simulink model "drone_position_estimate_discrete"  (R2020b)
settings: Solver=VariableStepAuto  StartTime=0.0  StopTime=30  RelTol=1e-3
values from neighbouring files (symbols this model uses):
  at = [1;0;-9.98]    [run_drone_estimate.m]
  cov_an = 1*eye(3)    [run_drone_estimate.m]
  cov_aw = 1*eye(3)    [run_drone_estimate.m]
  cov_gps = .01*eye(3)    [run_drone_estimate.m]
  F_discrete = F_discrete + (aux/factorial(i))    [run_drone_estimate.m]
  g = [0;0;-9.98]    [run_drone_estimate.m]
  h = 1    [run_drone_estimate.m]
  H_discrete = H    [run_drone_estimate.m]
  L = lqe(F, G, H, Q, R)    [run_drone_estimate.m]
  p0 = zeros(3,1)    [run_drone_estimate.m]
  Rm = eye(3)    [run_drone_estimate.m]
  v0 = zeros(3,1)    [run_drone_estimate.m]
  x0_observer = zeros(n, 1)    [run_drone_estimate.m]
settings Model: Creator=lucas  LastModifiedBy=lucas

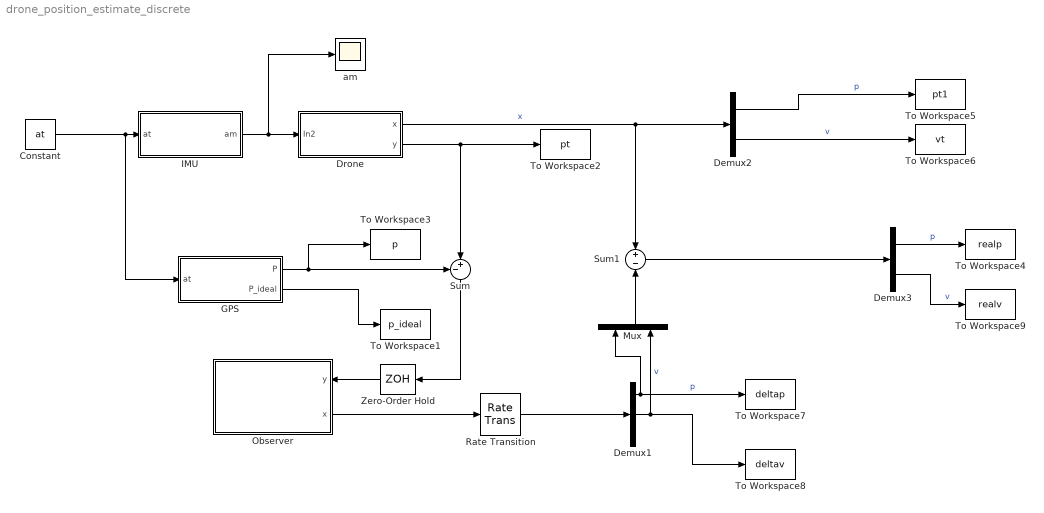
== system drone_position_estimate_discrete ==
  Constant : Constant  Value=at
  Demux1 : Demux  Outputs=3
  Demux2 : Demux  Outputs=2
  Demux3 : Demux  Outputs=2
  Drone : Subsystem
  GPS : Subsystem
  IMU : Subsystem
  Mux : Mux  Inputs=2
  Observer : Subsystem
      settings: PortSchema="{\"entries\":[{\"content\":{\"sides\":[{\"content\":{\"connectorIds\":[]},\"type\":\"ConnectorPlacement.EquallySpacedRectSide\",\"uuid\":\"b6dae28a-5485-44ef-84e6-2d14792229e7\"},{\"content\":{\"connectorIds\":[\"In1\",\"Out1\"],\"side\":\"RIGHT\"},\"type\":\"ConnectorPlacement.EquallySpacedRectSide\",\"uuid\":\"53a86c87-87d1-415f-9895-91b2b6ac7daf\"},{\"content\":{\"connectorIds\":[],\"side\":\"TOP\"},\"type\":\"ConnectorPlacement.EquallySpacedRectSide\",\"uuid\":\"c2916f3e-51bf-40f4-b6cd-eee6b60c38ec\"},{\"content\":{\"connectorIds\":[],\"side\":\"HIDDEN\"},\"type\":\"ConnectorPlacement.EquallySpacedRectSide\",\"uuid\":\"c85aafdf-e330-4d8d-a14a-206e12d7d836\"}]},\"type\":\"ConnectorPlacement.EquallySpacedConnector\",\"uuid\":\"08a8a426-31b9-42c2-8372-de3a4deaf2af\"}],\"packageUris\":[\"http://schema.mathworks.com/mf0/Connector/R2020b\"],\"version\":\"1.0\"}"
  Rate Transition : RateTransition  OutPortSampleTimeOpt=Inherit  OutPortSampleTimeMultiple=h_plant  OutPortSampleTime=h_plant
  Sum : Sum  Inputs=-+|
  Sum1 : Sum  Inputs=+|-
  To Workspace1 : ToWorkspace  VariableName=p_ideal  SaveFormat=Timeseries  SampleTime=-1
  To Workspace2 : ToWorkspace  VariableName=pt  SaveFormat=Timeseries  SampleTime=-1
  To Workspace3 : ToWorkspace  VariableName=p  SaveFormat=Timeseries  SampleTime=-1
  To Workspace4 : ToWorkspace  VariableName=realp  SaveFormat=Timeseries  SampleTime=-1
  To Workspace5 : ToWorkspace  VariableName=pt1  SaveFormat=Timeseries  SampleTime=-1
  To Workspace6 : ToWorkspace  VariableName=vt  SaveFormat=Timeseries  SampleTime=-1
  To Workspace7 : ToWorkspace  VariableName=deltap  SaveFormat=Timeseries  SampleTime=-1
  To Workspace8 : ToWorkspace  VariableName=deltav  SaveFormat=Timeseries  SampleTime=-1
  To Workspace9 : ToWorkspace  VariableName=realv  SaveFormat=Timeseries  SampleTime=-1
  Zero-Order Hold : ZeroOrderHold  SampleTime=h
  am : Scope
  wires:
  GPS/2(P_ideal) -> To Workspace1/1
  Constant/1 -> GPS/1(at), IMU/1(at)
  GPS/1(P) -> Sum/1, To Workspace3/1
  Demux1/1 -> Mux/1, To Workspace7/1  "p"
  IMU/1(am) -> am/1, Drone/1(In2)
  Demux1/2 -> Mux/2, To Workspace8/1  "v"
  Drone/1(x) -> Demux2/1, Sum1/1  "x"
  Demux2/2 -> To Workspace6/1  "v"
  Demux2/1 -> To Workspace5/1  "p"
  Drone/2(y) -> Sum/2, To Workspace2/1
  Zero-Order Hold/1 -> Observer/1(y)
  Sum/1 -> Zero-Order Hold/1
  Observer/1(x) -> Rate Transition/1
  Rate Transition/1 -> Demux1/1
  Sum1/1 -> Demux3/1
  Demux3/1 -> To Workspace4/1  "p"
  Demux3/2 -> To Workspace9/1  "v"
  Mux/1 -> Sum1/2

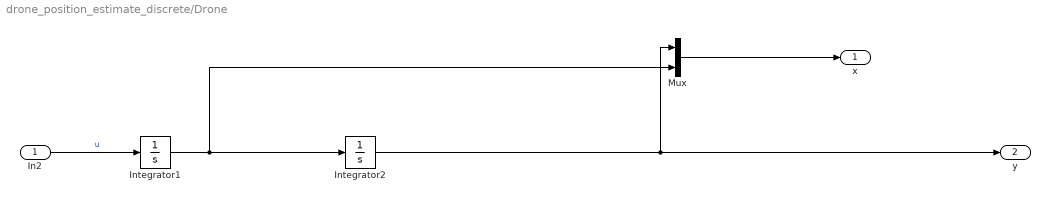
== system drone_position_estimate_discrete/Drone ==
  In2 : Inport
  Integrator1 : Integrator  InitialCondition=v0
  Integrator2 : Integrator  InitialCondition=p0
  Mux : Mux  Inputs=2
  x : Outport
  y : Outport  Port=2
  wires:
  In2/1 -> Integrator1/1  "u"
  Integrator1/1 -> Integrator2/1, Mux/2
  Integrator2/1 -> Mux/1, y/1
  Mux/1 -> x/1

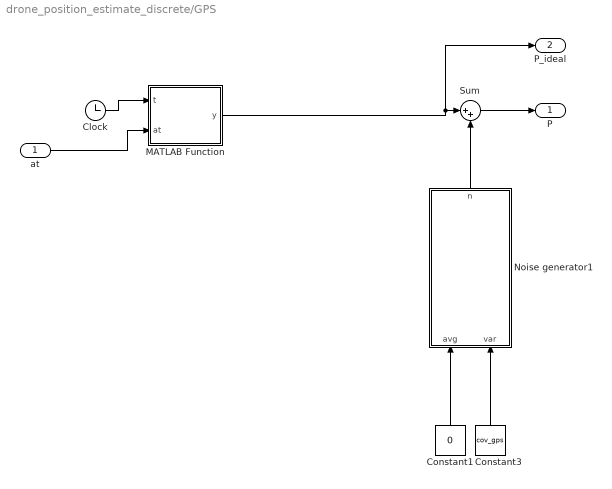
== system drone_position_estimate_discrete/GPS ==
  at : Inport
  Clock : Clock
  Constant1 : Constant  Value=0
  Constant3 : Constant  Value=cov_gps
  MATLAB Function : MATLAB Function  TreatAsAtomicUnit=on
  Noise generator1 : MATLAB Function  TreatAsAtomicUnit=on
  Sum : Sum  Inputs=|++
  P : Outport
  P_ideal : Outport  Port=2
  wires:
  Noise generator1/1(n) -> Sum/2
  Constant3/1 -> Noise generator1/2(var)
  Constant1/1 -> Noise generator1/1(avg)
  Sum/1 -> P/1
  Clock/1 -> MATLAB Function/1(t)
  MATLAB Function/1(y) -> P_ideal/1, Sum/1
  at/1 -> MATLAB Function/2(at)

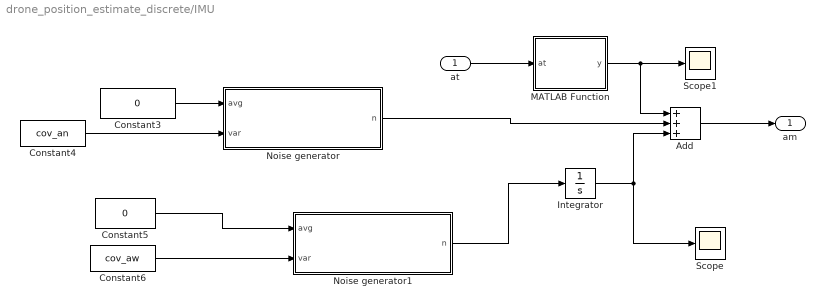
== system drone_position_estimate_discrete/IMU ==
  at : Inport
  Add : Sum  Inputs=+++
  Constant3 : Constant  Value=0  VectorParams1D=off
  Constant4 : Constant  Value=cov_an  VectorParams1D=off
  Constant5 : Constant  Value=0  VectorParams1D=off
  Constant6 : Constant  Value=cov_aw  VectorParams1D=off
  Integrator : Integrator
  MATLAB Function : MATLAB Function  TreatAsAtomicUnit=on
  Noise generator : MATLAB Function  TreatAsAtomicUnit=on
  Noise generator1 : MATLAB Function  TreatAsAtomicUnit=on
  Scope : Scope
  Scope1 : Scope
  am : Outport
  wires:
  Add/1 -> am/1
  Integrator/1 -> Scope/1, Add/3
  MATLAB Function/1(y) -> Scope1/1, Add/1
  Constant3/1 -> Noise generator/1(avg)
  Constant4/1 -> Noise generator/2(var)
  Noise generator/1(n) -> Add/2
  Constant6/1 -> Noise generator1/2(var)
  Constant5/1 -> Noise generator1/1(avg)
  Noise generator1/1(n) -> Integrator/1
  at/1 -> MATLAB Function/1(at)

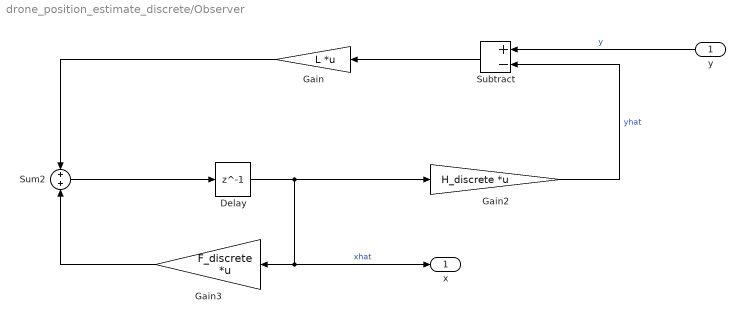
== system drone_position_estimate_discrete/Observer ==
  y : Inport
  Delay : Delay  DelayLength=1  InitialCondition=x0_observer
  Gain : Gain  Gain=L  Multiplication=Matrix(K*u) (u vector)
  Gain2 : Gain  Gain=H_discrete  Multiplication=Matrix(K*u) (u vector)
  Gain3 : Gain  Gain=F_discrete  Multiplication=Matrix(K*u) (u vector)
  Subtract : Sum  Inputs=+-
  Sum2 : Sum  Inputs=+|+
  x : Outport
  wires:
  Sum2/1 -> Delay/1
  Gain3/1 -> Sum2/2
  Delay/1 -> Gain3/1, x/1, Gain2/1  "xhat"
  y/1 -> Subtract/1  "y"
  Gain2/1 -> Subtract/2  "yhat"
  Subtract/1 -> Gain/1
  Gain/1 -> Sum2/1

== matlab function drone_position_estimate_discrete/IMU/Noise generator ==
  data: avg input; n output; var input
function n = generate_gaussian_noise(avg, var)
n = avg + var*randn(length(var), 1);

== matlab function drone_position_estimate_discrete/GPS/MATLAB Function ==
  data: t input; y output; v0 parameter; g parameter; Rm parameter; at input; p0 parameter
function y = gps_pos(t, v0, g, Rm, at, p0)
    accel = Rm*(at - g);
    y = zeros(3,1);
    for i = 1:3
        y(i) = p0(i) + (v0(i)*t) + (accel(i)*(t^2)/2);
    end

== matlab function drone_position_estimate_discrete/GPS/Noise generator1 ==
  data: avg input; n output; var input
function n = generate_gaussian_noise(avg, var)
n = avg + var*randn(length(var), 1);

== matlab function drone_position_estimate_discrete/IMU/MATLAB Function ==
  data: y output; Rm parameter; g parameter; at input
function y = fcn(Rm, g, at)
    y=Rm*(at-g);

== matlab function drone_position_estimate_discrete/IMU/Noise generator1 ==
  data: avg input; n output; var input
function n = generate_gaussian_noise(avg, var)
n = avg + var*randn(length(var), 1);
